simulink model "ZOP_Main"  (R2018b)
settings: Solver=FixedStepDiscrete  StartTime=0.0  StopTime=inf  FixedStep=0.01  RelTol=1e-3
PostLoadFcn:
  | if any(exist('dsrtsu_mdlpostloadfcn', 'file') ~= 0), dsrtsu_mdlpostloadfcn('Execute', bdroot); end
values from neighbouring files (symbols this model uses):
  k_ZOP_ALC_Ramp = 1.0    [ZOP_Func.sldd]
  k_ZOP_LS_ChangingDist = 5.0    [ZOP_Func.sldd]
  k_ZOP_LS_ChangingTime = 0.5    [ZOP_Func.sldd]
  k_ZOP_SpdLmt_Enable = 1.0    [ZOP_Func.sldd]
  k_ZOP_V2X_Enable = 1.0    [ZOP_Func.sldd]
  k_ZOP_VcTJA_Enable = 1.0    [ZOP_Func.sldd]
  k_ZOP_VoiceAct_Enable = 1.0    [ZOP_Func.sldd]
  MODE_ZOP_ACTIVE = 3.0    [ZOP_Func.sldd]
  MODE_ZOP_FINISH = 10.0    [ZOP_Func.sldd]
  MODE_ZOP_LC = 7.0    [ZOP_Func.sldd]
(part 1 of 2)
settings Model: DSRTSU_INTERNAL_RTI_VER=540  DSRTSU_INTERNAL_RTI_TYPE=rti1401  RTICANMMDATA=struct('GeneralSetupData',struct('modelroot','F:\DatabaseZO\08.Code\Model\ZOP_Integration','generalsettings',struct('filesettings',struct('destfolder',struct('Name','RTICANMM_FILES','Check',1),'buildfolder',struct('Name','.','Check',1),'AbsDestfolder',struct('Name','F:\DatabaseZO\08.Code\Model\ZOP_Integration\RTICANMM_FILES'),'AbsBuildfolder',struct('Name','F:\DatabaseZO\08.Code\Model\ZOP_Integration'))),'options',struct('addpaths',1,'rmpaths',1,'addtrcexclusion',logical(1),'cannavigator',struct('checkmonitoring',0),'show_usrtrc',0,'use_usrtrc',0),'advanced',struct('options',ones(1,100)),'MPSetup',{{}},'RTI',struct('Type','RTI1401','Ver','7.12','Date','02-May-2019'),'modelname','ZOP_Main','block','ZOP_Main'))  DSRTSU_INTERNAL_RTIFPGA=130  Creator=zjw  LastModifiedBy=zjw
settings OptimizationCC: BlockReduction=off  ConditionallyExecuteInputs=off  DefaultUnderspecifiedDataType=single  BufferReuse=off  EnhancedBackFolding=on  ExpressionFolding=off  PassReuseOutputArgsThreshold=0  LocalBlockOutputs=off  OptimizeBlockOrder=speed  DifferentSizesBufferReuse=on
settings DebuggingCC: ParameterTunabilityLossMsg=error
settings HardwareCC: ProdBitPerPointer=32  ProdBitPerSizeT=32  ProdBitPerPtrDiffT=32  ProdLargestAtomicInteger=Integer  ProdEndianess=BigEndian  ProdWordSize=32  ProdHWDeviceType=Custom Processor->Custom  TargetIntDivRoundTo=Zero  TargetEndianess=BigEndian  TargetHWDeviceType=Custom Processor->Custom
settings ModelReferenceCC: ModelReferenceNumInstancesAllowed=Single
settings SFSimCC: MATLABDynamicMemAlloc=off
settings RTWCC: SystemTargetFile=rti1401.tlc  MakeCommand=make_rti  TemplateMakefile=rti1401.tmf  Description=dSPACE DS1401 Hardware Platform  GenerateReport=on  LaunchReport=on
settings CodeAppCC: OperatorAnnotations=on
settings STFCustomTargetCC: ParMdlRefBuildCompliant=on  SystemTargetFile=rti1401.tlc
settings GRTTargetCC: TargetLangStandard=C89/C90 (ANSI)  CompOptLevelCompliant=off  ConcurrentExecutionCompliant=off  CombineOutputUpdateFcns=off  MatFileLogging=off  CPPClassGenCompliant=off  UseToolchainInfoCompliant=off

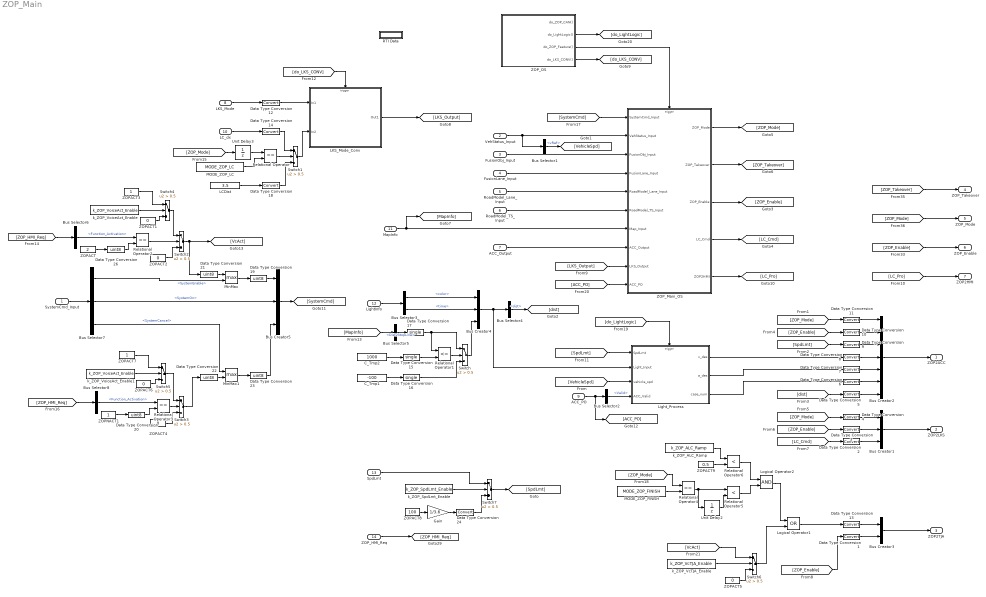
== system ZOP_Main ==
  SystemCmd_Input : Inport  OutDataTypeStr=Bus: SystemCmd_ST  BusOutputAsStruct=on
  VehStatus_Input : Inport  Port=2  OutDataTypeStr=Bus: VSI_VEHSTATE_ST  BusOutputAsStruct=on
  FusionObj_Input : Inport  Port=3  OutDataTypeStr=Bus: FUS_OBJ_OUTPUT_ST  BusOutputAsStruct=on
  FusionLane_Input : Inport  Port=4  OutDataTypeStr=Bus: FUS_LANE_OUTPUT_ST  BusOutputAsStruct=on
  RoadModel_Lane_Input : Inport  Port=5  OutDataTypeStr=Bus: LANEMODEL_OUTPUT_ST  BusOutputAsStruct=on
  RoadModel_TS_Input : Inport  Port=6  OutDataTypeStr=Bus: HWA_TARGETOBJECT_OUTPUT_ST  BusOutputAsStruct=on
  ACC_Output : Inport  Port=7  OutDataTypeStr=Bus: ACC_Status_ST  BusOutputAsStruct=on
  LKS_Mode : Inport  Port=8  BusOutputAsStruct=on
  ACC_PO : Inport  Port=9  OutDataTypeStr=Bus: ATS_PO_ST  BusOutputAsStruct=on
  LC_dx : Inport  Port=10  BusOutputAsStruct=on
  MapInfo : Inport  Port=11  OutDataTypeStr=Bus: MapInfo_ST  BusOutputAsStruct=on
  LightInfo : Inport  Port=12  OutDataTypeStr=Bus: Light_Info_ST  BusOutputAsStruct=on
  SpdLmt : Inport  Port=13  BusOutputAsStruct=on
  ZOP_HMI_Req : Inport  Port=14  OutDataTypeStr=Bus: ZOP_HMI_REQ  BusOutputAsStruct=on
  Bus Creator1 : BusCreator  Inputs=3  OutDataTypeStr=Bus: ZOP2LCK  NonVirtualBus=on
      settings: InheritFromInputs=off
  Bus Creator2 : BusCreator  Inputs=7  OutDataTypeStr=Bus: ZOP2ACC  NonVirtualBus=on
      settings: InheritFromInputs=off
  Bus Creator3 : BusCreator  Inputs=2  OutDataTypeStr=Bus: ZOP2TJA  NonVirtualBus=on
      settings: InheritFromInputs=off
  Bus Creator4 : BusCreator  Inputs=3  OutDataTypeStr=Bus: Light_Info_ST  NonVirtualBus=on
      settings: InheritFromInputs=off
  Bus Creator5 : BusCreator  Inputs=3  OutDataTypeStr=Bus: SystemCmd_ST  NonVirtualBus=on
      settings: InheritFromInputs=off
  Bus Selector1 : BusSelector  OutputSignals=vRef
  Bus Selector2 : BusSelector  OutputSignals=Valid
  Bus Selector3 : BusSelector  OutputSignals=color,time
  Bus Selector4 : BusSelector  OutputSignals=dist
  Bus Selector5 : BusSelector  OutputSignals=Dist2StopLine
  Bus Selector6 : BusSelector  OutputSignals=Function_Activation
  Bus Selector7 : BusSelector  OutputSignals=SystemEnable,SystemOn,SystemCancel
  Bus Selector8 : BusSelector  OutputSignals=Function_Activation
  C_Tmp1 : Constant  Value=-100
  C_Tmp2 : Constant  Value=1000
  Data Type Conversion{1..14,18,24} (16 alike) : DataTypeConversion
  Data Type Conversion15 : DataTypeConversion  OutDataTypeStr=single
  Data Type Conversion16 : DataTypeConversion  OutDataTypeStr=single
  Data Type Conversion17 : DataTypeConversion  OutDataTypeStr=single
  Data Type Conversion{19..23,26} (6 alike) : DataTypeConversion  OutDataTypeStr=uint8
  Gain : Gain  Gain=1/3.6
  LCDist : Constant  Value=3.5
  LKS_Mode_Conv : Subsystem
  Light_Process : Subsystem
  Logical Operator1 : Logic  Operator=OR  AllPortsSameDT=off  OutDataTypeStr=boolean
  Logical Operator2 : Logic  AllPortsSameDT=off  OutDataTypeStr=boolean
  MODE_ZOP_FINISH : Constant  Value=MODE_ZOP_FINISH
  MODE_ZOP_LC : Constant  Value=MODE_ZOP_LC
  MinMax : MinMax  Function=max  Inputs=2
  MinMax1 : MinMax  Function=max  Inputs=2
  RTI Data : Subsystem  Tag=struct('RTIDataServer',struct('RTIDataServerVs','2','RTIModelDescription','struct(''main'',''ZOP_Main'',''sub'','''',''isMp'',0)'))  LoadFcn="if exist('rtidc'), try,  rtidc('DataHostBlockClbLoad', gcbh); catch, disp(['Warning: ''LoadFcn'' for RTI Data block failed: ' lasterr]); end, end,"  mask(RTI_DATA_HOST){}
      mask help:
      | RTI Data Block.
      | This block is used by RTI to store internal model-dependent data.
      | Please keep this block on the root level of the model. Deleting this block will result in data loss.
      |
      | NEVER DELETE OR COPY THIS BLOCK!
      settings: CopyFcn="if exist('rtidc'), try,  rtidc('DataHostBlockClbCopy', gcbh); catch, disp(['Warning: ''CopyFcn'' for RTI Data block failed: ' lasterr]); end, end,"  DeleteFcn="if exist('rtidc'), try,  rtidc('DataHostBlockClbDelete', gcbh); catch, disp(['Warning: ''DeleteFcn'' for RTI Data block failed: ' lasterr]); end, end,"  ModelCloseFcn="if exist('rtidc'), try,  rtidc('DataHostBlockClbModelClose', gcbh); catch, disp(['Warning: ''ModelCloseFcn'' for RTI Data block failed: ' lasterr]); end, end,"  PreSaveFcn="if exist('rtidc'), try,  rtidc('DataHostBlockClbPreSave', gcbh); catch, disp(['Warning: ''PreSaveFcn'' for RTI Data block failed: ' lasterr]); end, end,"  PostSaveFcn="if exist('rtidc'), try,  rtidc('DataHostBlockClbPostSave', gcbh); catch, disp(['Warning: ''PostSaveFcn'' for RTI Data block failed: ' lasterr]); end, end,"  NameChangeFcn="if exist('rtidc'), try,  rtidc('DataHostBlockClbNameChange', gcbh); catch, disp(['Warning: ''NameChangeFcn'' for RTI Data block failed: ' lasterr]); end, end,"
      mask Help:
      | RTI Data Block.
      | This block is used by RTI to store internal model-dependent data.
      | Please keep this block on the root level of the model. Deleting this block will result in data loss.
      | 
      | NEVER DELETE OR COPY THIS BLOCK!
      mask Display:
      | text(0.5, 0.5, 'RTI Data', 'HorizontalAlignment', 'center');
      | plot([1 0]);
  Relational Operator{,2..4} (4 alike) : RelationalOperator  Operator===  OutDataTypeStr=boolean  RndMeth=Simplest
  Relational Operator1 : RelationalOperator  Operator=<=  OutDataTypeStr=boolean  RndMeth=Simplest
  Relational Operator5 : RelationalOperator  Operator=<  OutDataTypeStr=boolean  RndMeth=Simplest
  Relational Operator6 : RelationalOperator  Operator=<  OutDataTypeStr=boolean  RndMeth=Simplest
  Switch{,1..7} (8 alike) : Switch  Criteria=u2 > Threshold  Threshold=0.5
  Unit Delay2 : UnitDelay  SampleTime=-1
  Unit Delay3 : UnitDelay  SampleTime=-1
  ZOPACT : Constant  Value=2
  ZOPACT{1..2,4..6} (5 alike) : Constant  Value=0
  ZOPACT3 : Constant
  ZOPACT7 : Constant
  ZOPACT8 : Constant  Value=100
  ZOPACT9 : Constant  Value=0.5
  ZOPNACT1 : Constant
  ZOP_Main_OS : Subsystem
  ZOP_OS : Stateflow chart  TreatAsAtomicUnit=on
  k_ZOP_ALC_Ramp : Constant  Value=k_ZOP_ALC_Ramp
  k_ZOP_SpdLmt_Enable : Constant  Value=k_ZOP_SpdLmt_Enable
  k_ZOP_VcTJA_Enable : Constant  Value=k_ZOP_VcTJA_Enable
  k_ZOP_VoiceAct_Enable : Constant  Value=k_ZOP_VoiceAct_Enable
  k_ZOP_VoiceAct_Enable1 : Constant  Value=k_ZOP_VoiceAct_Enable
  ZOP2ACC : Outport  OutDataTypeStr=Bus: ZOP2ACC
  ZOP2LKS : Outport  Port=2  OutDataTypeStr=Bus: ZOP2LCK
  ZOP2TJA : Outport  Port=3  OutDataTypeStr=Bus: ZOP2TJA
  ZOP_Takeover : Outport  Port=4
  ZOP_Mode : Outport  Port=5
  ZOP_Enable : Outport  Port=6
  ZOP2HMI : Outport  Port=7  OutDataTypeStr=Bus: ZOP2HMI
  wires:
  ZOP_OS/3(do_ZOP_Feature()) -> ZOP_Main_OS/Trigger
  ZOP_Main_OS/1(ZOP_Mode) -> [ZOP_Mode]
  ZOP_Main_OS/2(ZOP_Takeover) -> [ZOP_Takeover]
  MapInfo/1 -> [MapInfo], ZOP_Main_OS/7(Map_Input)
  ZOP_OS/2(do_LightLogic()) -> [do_LightLogic]
  [do_LightLogic] -> Light_Process/Trigger
  VehStatus_Input/1 -> Bus Selector1/1, ZOP_Main_OS/2(VehStatus_Input)
  FusionObj_Input/1 -> ZOP_Main_OS/3(FusionObj_Input)
  FusionLane_Input/1 -> ZOP_Main_OS/4(FusionLane_Input)
  RoadModel_Lane_Input/1 -> ZOP_Main_OS/5(RoadModel_Lane_Input)
  RoadModel_TS_Input/1 -> ZOP_Main_OS/6(RoadModel_TS_Input)
  Bus Selector1/1 -> [VehicleSpd]  "<vRef>"
  [VehicleSpd] -> Light_Process/3(vehicle_spd)
  ACC_PO/1 -> [ACC_PO], Bus Selector2/1
  Bus Selector2/1 -> Light_Process/4(ACC_Valid)  "<Valid>"
  [ZOP_Mode] -> Data Type Conversion11/1
  [SpdLmt] -> Data Type Conversion9/1
  Bus Selector4/1 -> [dist]  "<dist>"
  Light_Process/1(v_des) -> Data Type Conversion8/1
  ZOP_Main_OS/3(ZOP_Enable) -> [ZOP_Enable]
  [ZOP_Enable] -> Data Type Conversion10/1
  [ZOP_Mode] -> Data Type Conversion4/1
  [ZOP_Enable] -> Data Type Conversion3/1
  ZOP_Main_OS/4(LC_Cmd) -> [LC_Cmd]
  [LC_Cmd] -> Data Type Conversion2/1
  Light_Process/2(a_des) -> Data Type Conversion7/1
  [dist] -> Data Type Conversion5/1
  Light_Process/3(case_num) -> Data Type Conversion6/1
  Data Type Conversion13/1 -> Bus Creator3/1
  [ZOP_Enable] -> Data Type Conversion1/1
  ACC_Output/1 -> ZOP_Main_OS/8(ACC_Output)
  [LKS_Output] -> ZOP_Main_OS/9(LKS_Output)
  Data Type Conversion1/1 -> Bus Creator3/2
  Data Type Conversion2/1 -> Bus Creator1/3
  Data Type Conversion3/1 -> Bus Creator1/2
  Data Type Conversion4/1 -> Bus Creator1/1
  Data Type Conversion5/1 -> Bus Creator2/7
  Data Type Conversion6/1 -> Bus Creator2/6
  Data Type Conversion7/1 -> Bus Creator2/5
  Data Type Conversion8/1 -> Bus Creator2/4
  Data Type Conversion9/1 -> Bus Creator2/3
  Data Type Conversion10/1 -> Bus Creator2/2
  Data Type Conversion11/1 -> Bus Creator2/1
  [SpdLmt] -> Light_Process/1(SpdLmt)
  LKS_Mode/1 -> Data Type Conversion12/1
  LC_dx/1 -> Data Type Conversion14/1
  LKS_Mode_Conv/1(Out1) -> [LKS_Output]
  ZOP_OS/4(do_LKS_CONV()) -> [do_LKS_CONV]
  [do_LKS_CONV] -> LKS_Mode_Conv/Trigger
  [ZOP_Takeover] -> ZOP_Takeover/1
  [ZOP_Mode] -> ZOP_Mode/1
  [ZOP_Enable] -> ZOP_Enable/1
  Data Type Conversion12/1 -> LKS_Mode_Conv/1(In1)
  Bus Creator2/1 -> ZOP2ACC/1
  Bus Creator1/1 -> ZOP2LKS/1
  Bus Creator3/1 -> ZOP2TJA/1
  LightInfo/1 -> Bus Selector3/1
  Bus Selector3/1 -> Bus Creator4/1  "<color>"
  Bus Selector3/2 -> Bus Creator4/2  "<time>"
  Bus Creator4/1 -> Light_Process/2(Light_Input), Bus Selector4/1
  Relational Operator1/1 -> Switch/2
  C_Tmp1/1 -> Data Type Conversion16/1
  Switch/1 -> Bus Creator4/3
  C_Tmp2/1 -> Data Type Conversion15/1
  Data Type Conversion15/1 -> Relational Operator1/2
  Data Type Conversion16/1 -> Switch/3
  ZOP_Main_OS/5(ZOP2HMI) -> [LC_Pro]
  [LC_Pro] -> ZOP2HMI/1
  [MapInfo] -> Bus Selector5/1
  Bus Selector5/1 -> Data Type Conversion17/1  "<Dist2StopLine>"
  Data Type Conversion17/1 -> Relational Operator1/1, Switch/1
  [ZOP_Mode] -> Unit Delay3/1
  MODE_ZOP_LC/1 -> Relational Operator/2
  Relational Operator/1 -> Switch1/2
  Switch1/1 -> LKS_Mode_Conv/2(In2)
  Data Type Conversion14/1 -> Switch1/1
  LCDist/1 -> Data Type Conversion18/1
  Unit Delay3/1 -> Relational Operator/1
  Data Type Conversion18/1 -> Switch1/3
  ZOP_HMI_Req/1 -> [ZOP_HMI_Req]
  [ZOP_HMI_Req] -> Bus Selector6/1
  SystemCmd_Input/1 -> Bus Selector7/1
  Bus Selector6/1 -> Relational Operator2/1  "<Function_Activation>"
  ZOPACT/1 -> Data Type Conversion26/1
  Data Type Conversion26/1 -> Relational Operator2/2
  Bus Selector7/1 -> MinMax/2  "<SystemEnable>"
  Bus Selector7/3 -> MinMax1/1  "<SystemCancel>"
  Data Type Conversion19/1 -> Bus Creator5/1
  MinMax/1 -> Data Type Conversion19/1
  Data Type Conversion20/1 -> Relational Operator3/2
  ZOPNACT1/1 -> Data Type Conversion20/1
  Bus Selector8/1 -> Relational Operator3/1  "<Function_Activation>"
  [ZOP_HMI_Req] -> Bus Selector8/1
  Relational Operator2/1 -> Switch2/2
  ZOPACT2/1 -> Switch2/3
  ZOPACT4/1 -> Switch3/3
  Switch2/1 -> Data Type Conversion21/1, [VcAct]
  Data Type Conversion21/1 -> MinMax/1
  Relational Operator3/1 -> Switch3/2
  Switch3/1 -> Data Type Conversion22/1
  Data Type Conversion22/1 -> MinMax1/2
  MinMax1/1 -> Data Type Conversion23/1
  Bus Creator5/1 -> [SystemCmd]
  [SystemCmd] -> ZOP_Main_OS/1(SystemCmd_Input)
  MODE_ZOP_FINISH/1 -> Relational Operator4/2
  [ZOP_Mode] -> Relational Operator4/1
  Bus Selector7/2 -> Bus Creator5/2  "<SystemOn>"
  Data Type Conversion23/1 -> Bus Creator5/3
  [ACC_PO] -> ZOP_Main_OS/10(ACC_PO)
  k_ZOP_VoiceAct_Enable/1 -> Switch4/2
  ZOPACT3/1 -> Switch4/1
  ZOPACT1/1 -> Switch4/3
  Switch4/1 -> Switch2/1
  ZOPACT6/1 -> Switch5/3
  k_ZOP_VoiceAct_Enable1/1 -> Switch5/2
  ZOPACT7/1 -> Switch5/1
  Switch5/1 -> Switch3/1
  Logical Operator1/1 -> Data Type Conversion13/1
  Switch6/1 -> Logical Operator1/2
  k_ZOP_VcTJA_Enable/1 -> Switch6/2
  ZOPACT5/1 -> Switch6/3
  [VcAct] -> Switch6/1
  SpdLmt/1 -> Switch7/1
  ZOPACT8/1 -> Gain/1
  k_ZOP_SpdLmt_Enable/1 -> Switch7/2
  Switch7/1 -> [SpdLmt]
  Gain/1 -> Data Type Conversion24/1
  Data Type Conversion24/1 -> Switch7/3
  Relational Operator4/1 -> Unit Delay2/1, Relational Operator5/1
  Unit Delay2/1 -> Relational Operator5/2
  Logical Operator2/1 -> Logical Operator1/1
  Relational Operator5/1 -> Logical Operator2/2
  Relational Operator6/1 -> Logical Operator2/1
  k_ZOP_ALC_Ramp/1 -> Relational Operator6/1
  ZOPACT9/1 -> Relational Operator6/2

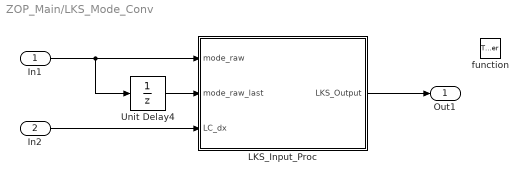
== system ZOP_Main/LKS_Mode_Conv ==
  In1 : Inport
  In2 : Inport  Port=2
  function : TriggerPort  TriggerType=function-call  VariantControl=Variant
  LKS_Input_Proc : MATLAB Function  TreatAsAtomicUnit=on
  Unit Delay4 : UnitDelay  SampleTime=-1
  Out1 : Outport
  wires:
  In1/1 -> LKS_Input_Proc/1(mode_raw), Unit Delay4/1
  Unit Delay4/1 -> LKS_Input_Proc/2(mode_raw_last)
  In2/1 -> LKS_Input_Proc/3(LC_dx)
  LKS_Input_Proc/1(LKS_Output) -> Out1/1

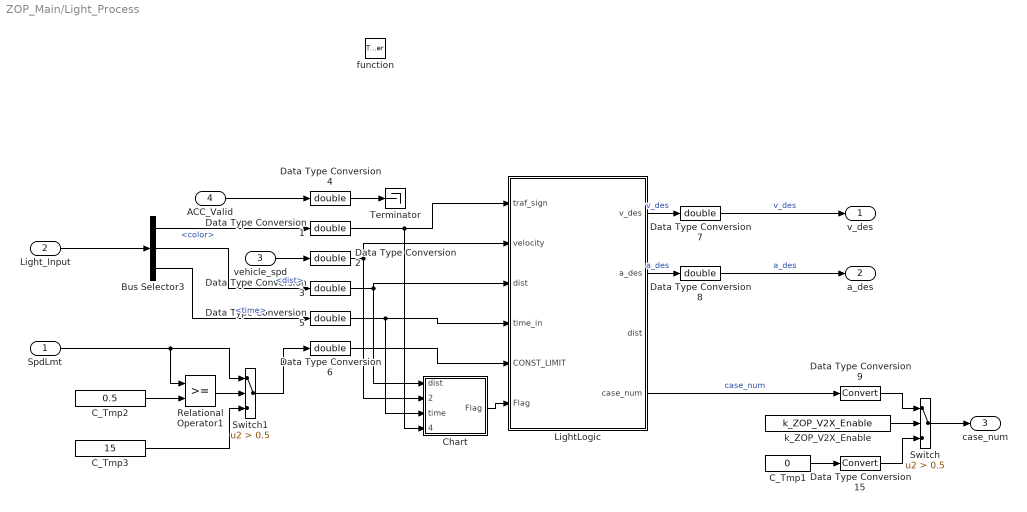
== system ZOP_Main/Light_Process ==
  SpdLmt : Inport  BusOutputAsStruct=on
  Light_Input : Inport  Port=2  OutDataTypeStr=Bus: Light_Info_ST  BusOutputAsStruct=on
  vehicle_spd : Inport  Port=3  BusOutputAsStruct=on
  ACC_Valid : Inport  Port=4  BusOutputAsStruct=on
  function : TriggerPort  TriggerType=function-call  VariantControl=Variant
  Bus Selector3 : BusSelector  OutputSignals=color,dist,time
  C_Tmp1 : Constant  Value=0
  C_Tmp2 : Constant  Value=0.5
  C_Tmp3 : Constant  Value=15
  Chart : Stateflow chart  TreatAsAtomicUnit=on
  Data Type Conversion{1..8} (8 alike) : DataTypeConversion  OutDataTypeStr=double
  Data Type Conversion15 : DataTypeConversion
  Data Type Conversion9 : DataTypeConversion
  LightLogic : MATLAB Function  TreatAsAtomicUnit=on
  Relational Operator1 : RelationalOperator  OutDataTypeStr=boolean  RndMeth=Simplest
  Switch : Switch  Criteria=u2 > Threshold  Threshold=0.5
  Switch1 : Switch  Criteria=u2 > Threshold  Threshold=0.5
  Terminator : Terminator
  k_ZOP_V2X_Enable : Constant  Value=k_ZOP_V2X_Enable
  v_des : Outport
  a_des : Outport  Port=2
  case_num : Outport  Port=3
  wires:
  Relational Operator1/1 -> Switch1/2
  C_Tmp2/1 -> Relational Operator1/2
  C_Tmp3/1 -> Switch1/3
  SpdLmt/1 -> Relational Operator1/1, Switch1/1
  LightLogic/2(a_des) -> Data Type Conversion8/1  "a_des"
  Bus Selector3/2 -> Data Type Conversion3/1  "<dist>"
  Data Type Conversion9/1 -> Switch/1
  Data Type Conversion3/1 -> Chart/1(dist), LightLogic/3("dist ")
  Switch/1 -> case_num/1
  Data Type Conversion1/1 -> Chart/4(traf_sign), LightLogic/1(traf_sign)
  Switch1/1 -> Data Type Conversion6/1
  LightLogic/4(case_num) -> Data Type Conversion9/1  "case_num"
  Data Type Conversion6/1 -> LightLogic/5(CONST_LIMIT)
  Data Type Conversion2/1 -> Chart/2(velocity), LightLogic/2(velocity)
  Bus Selector3/1 -> Data Type Conversion1/1  "<color>"
  Data Type Conversion8/1 -> a_des/1  "a_des"
  Chart/1(Flag) -> LightLogic/6(Flag)
  Bus Selector3/3 -> Data Type Conversion5/1  "<time>"
  ACC_Valid/1 -> Data Type Conversion4/1
  k_ZOP_V2X_Enable/1 -> Switch/2
  Data Type Conversion5/1 -> Chart/3(time), LightLogic/4(time_in)
  Data Type Conversion7/1 -> v_des/1  "v_des"
  C_Tmp1/1 -> Data Type Conversion15/1
  LightLogic/1(v_des) -> Data Type Conversion7/1  "v_des"
  vehicle_spd/1 -> Data Type Conversion2/1
  Data Type Conversion15/1 -> Switch/3
  Data Type Conversion4/1 -> Terminator/1
  Light_Input/1 -> Bus Selector3/1

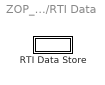
== system ZOP_Main/RTI Data ==
  RTI Data Store : Subsystem  Tag="struct('private',struct('version',struct('dsVer',uint32(2),'dsVerCreation',uint32(2),'RTI',struct('ver','7.12','type','RTI1401')),'access',struct('type','Model','isPerm',1,'created',['30-Dec-2020 11:01:12'],'modified',['10-Mar-2021 09:22:38'],'location','')),'public',struct('main',struct('data',[]),'sub',struct('name',{{'ZOP_Main'}},'data',{{struct('TH',struct('thTaskInfo',struct('taskType',{'TIMER','HWINT','TMRINT','SWINT','GLINT'},'tasksNumOf',{1,0,0,0,0},'srcIds',{{'TIMERA'},{},{},{},{}},'taskNames',{{['Timer Task 1']},{},{},{},{}})),'th_tc',struct('dataType','TASK','taskGroupId','','taskGroupList',{{}},'taskSchedulingPolicy','FCFS','taskType','TIMER','blkh',-1,'srcId','TIMERA','srcSgnName',['Timer A interrupt'],'srcCpuName','','taskName',['Timer Task 1  [0.01] s'],'taskNameDisplayExt','','smplTime',0.01,'smplTimeOffs',0,'hasFixedPriority',0,'priority',1,'hasFixedOvc',0,'ovcType',3,'ovcMax',1),'tc_th',struct('dataType','TASK','taskGroupId','','taskGroupList',{{}},'taskSchedulingPolicy','FCFS','taskType','TIMER','blkh',-1,'srcId','TIMERA','srcSgnName',['Timer A interrupt'],'srcCpuName','','taskName',['Timer Task 1  [0.01] s'],'taskNameDisplayExt','','smplTime',0.01,'smplTimeOffs',0,'hasFixedPriority',0,'priority',1,'hasFixedOvc',0,'ovcType',3,'ovcMax',1))}})))"  mask(RTI_DATA_STORE){}
      mask help:
      | RTI Data Store Block. This block is used by RTI to store internal model dependent data. Deleting this block will result in data loss.
      |
      | NEVER DELETE, COPY, OR MODIFY THIS BLOCK!
      mask Help:
      | RTI Data Store Block. This block is used by RTI to store internal model dependent data. Deleting this block will result in data loss.
      | 
      | NEVER DELETE, COPY, OR MODIFY THIS BLOCK!
      mask Display: text(0.5, 0.5, ' ', 'HorizontalAlignment', 'center');

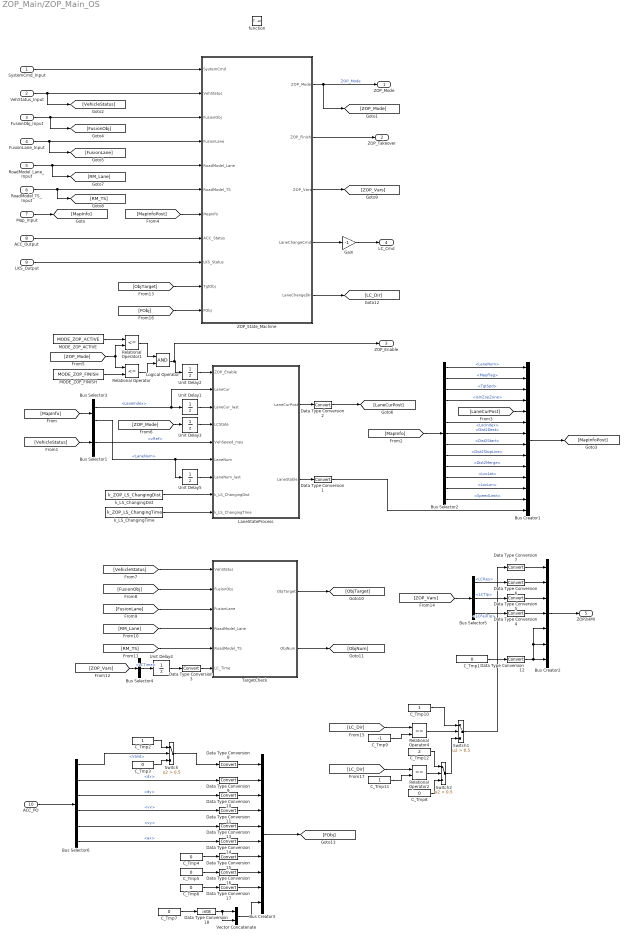
== system ZOP_Main/ZOP_Main_OS ==
  SystemCmd_Input : Inport  OutDataTypeStr=Bus: SystemCmd_ST  BusOutputAsStruct=on
  VehStatus_Input : Inport  Port=2  OutDataTypeStr=Bus: VSI_VEHSTATE_ST  BusOutputAsStruct=on
  FusionObj_Input : Inport  Port=3  OutDataTypeStr=Bus: FUS_OBJ_OUTPUT_ST  BusOutputAsStruct=on
  FusionLane_Input : Inport  Port=4  OutDataTypeStr=Bus: FUS_LANE_OUTPUT_ST  BusOutputAsStruct=on
  RoadModel_Lane_Input : Inport  Port=5  OutDataTypeStr=Bus: LANEMODEL_OUTPUT_ST  BusOutputAsStruct=on
  RoadModel_TS_Input : Inport  Port=6  OutDataTypeStr=Bus: HWA_TARGETOBJECT_OUTPUT_ST  BusOutputAsStruct=on
  Map_Input : Inport  Port=7  OutDataTypeStr=Bus: MapInfo_ST  BusOutputAsStruct=on
  ACC_Output : Inport  Port=8  OutDataTypeStr=Bus: ACC_Status_ST  BusOutputAsStruct=on
  LKS_Output : Inport  Port=9  OutDataTypeStr=Bus: LKS_Status_ST  BusOutputAsStruct=on
  ACC_PO : Inport  Port=10  OutDataTypeStr=Bus: ATS_PO_ST  BusOutputAsStruct=on
  function : TriggerPort  TriggerType=function-call  VariantControl=Variant
  Bus Creator1 : BusCreator  Inputs=14  OutDataTypeStr=Bus: MapInfo_ST_Post  NonVirtualBus=on
      settings: InheritFromInputs=off
  Bus Creator2 : BusCreator  Inputs=7  OutDataTypeStr=Bus: ZOP2HMI  NonVirtualBus=on
      settings: InheritFromInputs=off
  Bus Creator3 : BusCreator  Inputs=10  OutDataTypeStr=Bus: ZOP_Object_ST  NonVirtualBus=on
      settings: InheritFromInputs=off
  Bus Selector1 : BusSelector  OutputSignals=vRef
  Bus Selector2 : BusSelector  OutputSignals=LaneNum,MapFlag,TgtSpd,isInZopZone,LaneIndex,LocIndex,Dist2Dest,Dist2Start,Dist2StopLine,Dist2Merge,LocLat,LocLon,SpeedLimit
  Bus Selector3 : BusSelector  OutputSignals=LaneIndex,LaneNum
  Bus Selector4 : BusSelector  OutputSignals=LCTime
  Bus Selector5 : BusSelector  OutputSignals=LCRes,LCTip,LCFailTip
  Bus Selector6 : BusSelector  OutputSignals=Valid,dx,dy,vx,vy,ax
  C_Tmp{1,3..8} (7 alike) : Constant  Value=0
  C_Tmp10 : Constant
  C_Tmp11 : Constant
  C_Tmp12 : Constant  Value=2
  C_Tmp2 : Constant
  C_Tmp9 : Constant  Value=-1
  Data Type Conversion{1..17} (17 alike) : DataTypeConversion
  Data Type Conversion18 : DataTypeConversion  OutDataTypeStr=int8
  Gain : Gain  Gain=-1
  LaneStateProcess : Stateflow chart  TreatAsAtomicUnit=on
  Logical Operator : Logic  AllPortsSameDT=off  OutDataTypeStr=boolean
  MODE_ZOP_ACTIVE : Constant  Value=MODE_ZOP_ACTIVE
  MODE_ZOP_FINISH : Constant  Value=MODE_ZOP_FINISH
  Relational Operator : RelationalOperator  Operator=<=  OutDataTypeStr=boolean  RndMeth=Simplest
  Relational Operator1 : RelationalOperator  Operator=<=  OutDataTypeStr=boolean  RndMeth=Simplest
  Relational Operator2 : RelationalOperator  Operator===  OutDataTypeStr=boolean  RndMeth=Simplest
  Relational Operator4 : RelationalOperator  Operator===  OutDataTypeStr=boolean  RndMeth=Simplest
  Switch : Switch  Criteria=u2 > Threshold  Threshold=0.5
  Switch1 : Switch  Criteria=u2 > Threshold  Threshold=0.5
  Switch2 : Switch  Criteria=u2 > Threshold  Threshold=0.5
  TargetCheck : Stateflow chart  TreatAsAtomicUnit=on
  Unit Delay{1..5} (5 alike) : UnitDelay  SampleTime=-1
  Vector Concatenate : Concatenate
  ZOP_State_Machine : Stateflow chart  TreatAsAtomicUnit=on
  k_LS_ChangingDist : Constant  Value=k_ZOP_LS_ChangingDist
  k_LS_ChangingTime : Constant  Value=k_ZOP_LS_ChangingTime
  ZOP_Mode : Outport
  ZOP_Takeover : Outport  Port=2
  ZOP_Enable : Outport  Port=3
  LC_Cmd : Outport  Port=4
  ZOP2HMI : Outport  Port=5  OutDataTypeStr=Bus: ZOP2HMI
  wires:
  SystemCmd_Input/1 -> ZOP_State_Machine/1(SystemCmd)
  VehStatus_Input/1 -> [VehicleStatus], ZOP_State_Machine/2(VehStatus)
  FusionObj_Input/1 -> [FusionObj], ZOP_State_Machine/3(FusionObj)
  FusionLane_Input/1 -> [FusionLane], ZOP_State_Machine/4(FusionLane)
  RoadModel_Lane_Input/1 -> [RM_Lane], ZOP_State_Machine/5(RoadModel_Lane)
  RoadModel_TS_Input/1 -> [RM_TS], ZOP_State_Machine/6(RoadModel_TS)
  Map_Input/1 -> [MapInfo]
  ACC_Output/1 -> ZOP_State_Machine/8(ACC_Status)
  LKS_Output/1 -> ZOP_State_Machine/9(LKS_Status)
  ZOP_State_Machine/3(ZOP_Vars) -> [ZOP_Vars]
  ZOP_State_Machine/1(ZOP_Mode) -> ZOP_Mode/1, [ZOP_Mode]  "ZOP_Mode"
  ZOP_State_Machine/2(ZOP_Finish) -> ZOP_Takeover/1
  Bus Selector3/1 -> LaneStateProcess/2(LaneCur), Unit Delay1/1  "<LaneIndex>"
  Unit Delay1/1 -> LaneStateProcess/3(LaneCur_last)
  Unit Delay2/1 -> LaneStateProcess/1(ZOP_Enable)
  Unit Delay5/1 -> LaneStateProcess/7(LaneNum_last)
  Data Type Conversion2/1 -> [LaneCurPost]
  Bus Selector3/2 -> Unit Delay5/1, LaneStateProcess/6(LaneNum)  "<LaneNum>"
  Bus Selector1/1 -> LaneStateProcess/5(VehSpeed_mps)  "<vRef>"
  LaneStateProcess/1(LaneCurPost) -> Data Type Conversion2/1
  LaneStateProcess/2(LaneStable) -> Data Type Conversion1/1
  k_LS_ChangingDist/1 -> LaneStateProcess/8(k_LS_ChangingDist)
  [MapInfo] -> Bus Selector3/1
  [VehicleStatus] -> Bus Selector1/1
  k_LS_ChangingTime/1 -> LaneStateProcess/9(k_LS_ChangingTime)
  Bus Creator1/1 -> [MapInfoPost]
  [MapInfo] -> Bus Selector2/1
  [MapInfoPost] -> ZOP_State_Machine/7(MapInfo)
  [ZOP_Mode] -> Relational Operator1/2, Relational Operator/1
  MODE_ZOP_FINISH/1 -> Relational Operator/2
  MODE_ZOP_ACTIVE/1 -> Relational Operator1/1
  Relational Operator1/1 -> Logical Operator/1
  Relational Operator/1 -> Logical Operator/2
  Logical Operator/1 -> ZOP_Enable/1, Unit Delay2/1
  [ZOP_Mode] -> Unit Delay3/1
  Unit Delay3/1 -> LaneStateProcess/4(LCState)
  [VehicleStatus] -> TargetCheck/1(VehStatus)
  [FusionObj] -> TargetCheck/2(FusionObj)
  [FusionLane] -> TargetCheck/3(FusionLane)
  [RM_Lane] -> TargetCheck/4(RoadModel_Lane)
  [RM_TS] -> TargetCheck/5(RoadModel_TS)
  [ZOP_Vars] -> Bus Selector4/1
  Bus Selector4/1 -> Unit Delay4/1  "<LCTime>"
  TargetCheck/1(ObjTarget) -> [ObjTarget]
  [ObjTarget] -> ZOP_State_Machine/10(TgtObj)
  TargetCheck/2(ObjNum) -> [ObjNum]
  Unit Delay4/1 -> Data Type Conversion3/1
  ZOP_State_Machine/4(LaneChangeCmd) -> Gain/1
  Gain/1 -> LC_Cmd/1
  Data Type Conversion3/1 -> TargetCheck/6(LC_Time)
  ZOP_State_Machine/5(LaneChangeDir) -> [LC_Dir]
  Bus Selector2/1 -> Bus Creator1/1  "<LaneNum>"
  Bus Selector2/2 -> Bus Creator1/2  "<MapFlag>"
  Bus Selector2/3 -> Bus Creator1/3  "<TgtSpd>"
  Bus Selector2/4 -> Bus Creator1/4  "<isInZopZone>"
  Bus Selector2/6 -> Bus Creator1/6  "<LocIndex>"
  Bus Selector2/7 -> Bus Creator1/7  "<Dist2Dest>"
  Bus Selector2/8 -> Bus Creator1/8  "<Dist2Start>"
  Bus Selector2/9 -> Bus Creator1/9  "<Dist2StopLine>"
  Bus Selector2/10 -> Bus Creator1/10  "<Dist2Merge>"
  Bus Selector2/11 -> Bus Creator1/11  "<LocLat>"
  Bus Selector2/12 -> Bus Creator1/12  "<LocLon>"
  Bus Selector2/13 -> Bus Creator1/13  "<SpeedLimit>"
  [LaneCurPost] -> Bus Creator1/5
  Data Type Conversion1/1 -> Bus Creator1/14
  [ZOP_Vars] -> Bus Selector5/1
  Switch1/1 -> Data Type Conversion7/1
  Bus Selector5/1 -> Data Type Conversion6/1  "<LCRes>"
  Bus Selector5/3 -> Data Type Conversion4/1  "<LCFailTip>"
  Bus Creator2/1 -> ZOP2HMI/1
  C_Tmp1/1 -> Data Type Conversion12/1
  Data Type Conversion12/1 -> Bus Creator2/6, Bus Creator2/5, Bus Creator2/7
  Bus Selector5/2 -> Data Type Conversion5/1  "<LCTip>"
  Data Type Conversion4/1 -> Bus Creator2/4
  Data Type Conversion5/1 -> Bus Creator2/3
  Data Type Conversion6/1 -> Bus Creator2/2
  Data Type Conversion7/1 -> Bus Creator2/1
  ACC_PO/1 -> Bus Selector6/1
  Bus Selector6/2 -> Data Type Conversion9/1  "<dx>"
  Bus Selector6/3 -> Data Type Conversion10/1  "<dy>"
  Bus Selector6/4 -> Data Type Conversion11/1  "<vx>"
  Bus Selector6/5 -> Data Type Conversion13/1  "<vy>"
  Bus Selector6/6 -> Data Type Conversion14/1  "<ax>"
  Data Type Conversion8/1 -> Bus Creator3/1
  Data Type Conversion9/1 -> Bus Creator3/2
  Data Type Conversion10/1 -> Bus Creator3/3
  Data Type Conversion11/1 -> Bus Creator3/4
  Data Type Conversion13/1 -> Bus Creator3/5
  Data Type Conversion14/1 -> Bus Creator3/6
  Bus Selector6/1 -> Switch/2  "<Valid>"
  C_Tmp3/1 -> Switch/3
  C_Tmp2/1 -> Switch/1
  Switch/1 -> Data Type Conversion8/1
  [FObj] -> ZOP_State_Machine/11(FObj)
  Bus Creator3/1 -> [FObj]
  Data Type Conversion15/1 -> Bus Creator3/7
  C_Tmp4/1 -> Data Type Conversion15/1
  C_Tmp5/1 -> Data Type Conversion16/1
  Data Type Conversion16/1 -> Bus Creator3/8
  C_Tmp6/1 -> Data Type Conversion17/1
  Data Type Conversion17/1 -> Bus Creator3/9
  C_Tmp7/1 -> Data Type Conversion18/1
  Data Type Conversion18/1 -> Vector Concatenate/2, Vector Concatenate/1
  Vector Concatenate/1 -> Bus Creator3/10
  [LC_Dir] -> Relational Operator4/1
  C_Tmp9/1 -> Relational Operator4/2
  Relational Operator4/1 -> Switch1/2
  C_Tmp10/1 -> Switch1/1
  C_Tmp11/1 -> Relational Operator2/2
  [LC_Dir] -> Relational Operator2/1
  Relational Operator2/1 -> Switch2/2
  C_Tmp8/1 -> Switch2/3
  C_Tmp12/1 -> Switch2/1
  Switch2/1 -> Switch1/3

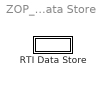
== system ZOP_Main/RTI Data/RTI Data Store ==
  RTI Data Store : Subsystem  mask(RTI_DATA_STORE){}
      mask help:
      | RTI Data Store Block. This block is used by RTI to store internal model dependent data. Deleting this block will result in data loss.
      |
      | NEVER DELETE, COPY, OR MODIFY THIS BLOCK!
      mask Help:
      | RTI Data Store Block. This block is used by RTI to store internal model dependent data. Deleting this block will result in data loss.
      | 
      | NEVER DELETE, COPY, OR MODIFY THIS BLOCK!
      mask Display: text(0.5, 0.5, ' ', 'HorizontalAlignment', 'center');

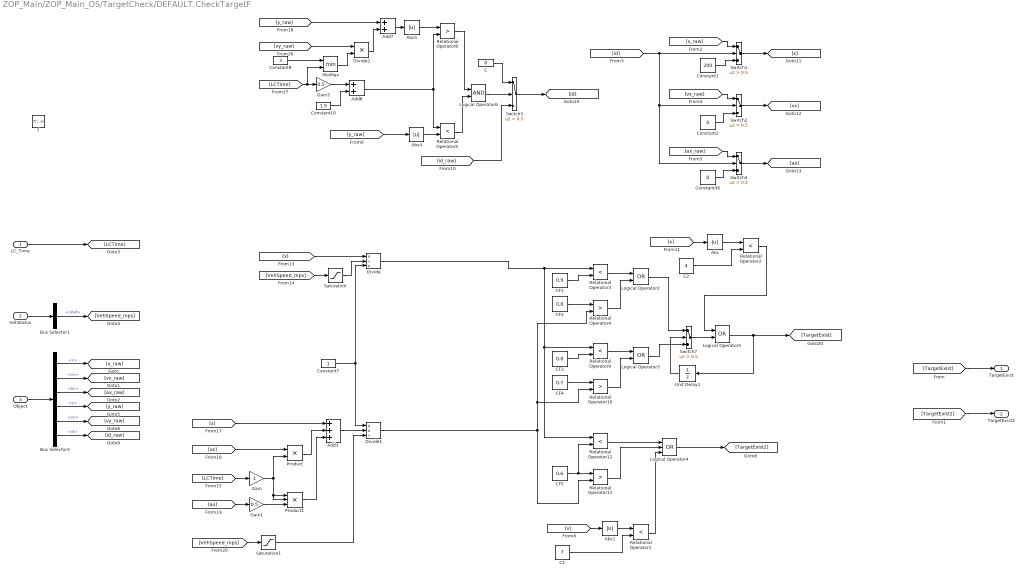
== system ZOP_Main/ZOP_Main_OS/TargetCheck/DEFAULT.CheckTargetF ==
  LC_Time : Inport  OutDataTypeStr=double
  VehStatus : Inport  Port=2  OutDataTypeStr=Bus: VSI_VEHSTATE_ST
  Object : Inport  Port=3  OutDataTypeStr=Bus: ZOP_Object_ST
  f : TriggerPort  TriggerType=function-call  VariantControl=(inherit)
      settings: CopyFcn=Stateflow.SLINSF.SimulinkMan.removeBlockPreDeleteFcn  PreDeleteFcn=Stateflow.SLINSF.SimulinkMan.unsafePredeleteFcn
  Abs{,1,4..5} (4 alike) : Abs
  Add3 : Sum  Inputs=+++
  Add6 : Sum
  Add7 : Sum
  Bus Selector1 : BusSelector  OutputSignals=vRef
  Bus Selector3 : BusSelector  OutputSignals=x,vx,ax,y,vy,id
  C : Constant  Value=0
  C1 : Constant  Value=7
  C2 : Constant  Value=4
  CF1 : Constant  Value=0.9
  CF2 : Constant  Value=0.8
  CF3 : Constant  Value=0.8
  CF4 : Constant  Value=0.7
  CF5 : Constant  Value=0.6
  Constant1 : Constant  Value=200
  Constant10 : Constant  Value=1.5
  Constant2 : Constant  Value=0
  Constant36 : Constant  Value=0
  Constant7 : Constant
  Constant9 : Constant  Value=3
  Divide : Product  Inputs=*/*
  Divide1 : Product  Inputs=**/
  Divide2 : Product  Inputs=**
  Gain : Gain
  Gain1 : Gain  Gain=0.5
  Gain3 : Gain  Gain=0.5
  Logical Operator2 : Logic  Operator=OR  AllPortsSameDT=off  OutDataTypeStr=boolean
  Logical Operator3 : Logic  Operator=OR  AllPortsSameDT=off  OutDataTypeStr=boolean
  Logical Operator4 : Logic  Operator=OR  Inputs=3  AllPortsSameDT=off  OutDataTypeStr=boolean
  Logical Operator5 : Logic  Operator=OR  AllPortsSameDT=off  OutDataTypeStr=boolean
  Logical Operator6 : Logic  AllPortsSameDT=off  OutDataTypeStr=boolean
  MinMax : MinMax  Inputs=2
  Product : Product
  Product1 : Product  Inputs=3
  Relational Operator{1..3,5,9,12} (6 alike) : RelationalOperator  Operator=<  RndMeth=Nearest
  Relational Operator{4,8,10..11} (4 alike) : RelationalOperator  Operator=>  RndMeth=Nearest
  Saturation : Saturate  UpperLimit=100  LowerLimit=0.1
  Saturation1 : Saturate  UpperLimit=100  LowerLimit=0.1
  Switch{1..4,7} (5 alike) : Switch  Criteria=u2 > Threshold  Threshold=0.5
  Unit Delay1 : UnitDelay  SampleTime=-1
  TargetExist : Outport
  TargetExist2 : Outport  Port=2
  wires:
  Abs1/1 -> Relational Operator1/1
  C1/1 -> Relational Operator1/2
  CF1/1 -> Relational Operator3/2
  Relational Operator1/1 -> Logical Operator4/3
  Relational Operator2/1 -> Logical Operator5/1
  [vx] -> Product/1
  [x] -> Abs/1
  [x] -> Abs1/1
  Switch7/1 -> Logical Operator5/2
  [ax] -> Gain1/1
  Logical Operator3/1 -> Switch7/3
  Logical Operator2/1 -> Switch7/1
  Relational Operator11/1 -> Logical Operator4/2
  Relational Operator10/1 -> Logical Operator3/2
  Gain1/1 -> Product1/3
  Divide1/1 -> Relational Operator11/2, Relational Operator4/2, Relational Operator10/2
  Relational Operator9/1 -> Logical Operator3/1
  Logical Operator4/1 -> [TargetExist2]
  Product1/1 -> Add3/3
  Add3/1 -> Divide1/2
  CF5/1 -> Relational Operator11/1, Relational Operator12/2
  Relational Operator3/1 -> Logical Operator2/1
  CF4/1 -> Relational Operator10/1
  [LCTime] -> Gain/1
  Unit Delay1/1 -> Switch7/2
  [x] -> Divide/1
  Constant7/1 -> Divide/3, Divide1/1
  C2/1 -> Relational Operator2/2
  Logical Operator5/1 -> [TargetExist], Unit Delay1/1
  [x] -> Add3/1
  [VehSpeed_mps] -> Saturation1/1
  Product/1 -> Add3/2
  Abs/1 -> Relational Operator2/1
  CF3/1 -> Relational Operator9/2
  CF2/1 -> Relational Operator4/1
  Relational Operator4/1 -> Logical Operator2/2
  Divide/1 -> Relational Operator12/1, Relational Operator9/1, Relational Operator3/1
  Gain/1 -> Product1/2, Product1/1, Product/2
  Saturation1/1 -> Divide1/3
  Relational Operator12/1 -> Logical Operator4/1
  Saturation/1 -> Divide/2
  [VehSpeed_mps] -> Saturation/1
  [TargetExist] -> TargetExist/1
  [TargetExist2] -> TargetExist2/1
  Object/1 -> Bus Selector3/1
  Bus Selector3/1 -> [x_raw]  "<x>"
  Bus Selector3/2 -> [vx_raw]  "<vx>"
  Bus Selector3/3 -> [ax_raw]  "<ax>"
  LC_Time/1 -> [LCTime]
  VehStatus/1 -> Bus Selector1/1
  Bus Selector1/1 -> [VehSpeed_mps]  "<vRef>"
  [id_raw] -> Switch3/3
  Relational Operator5/1 -> Logical Operator6/2
  [y_raw] -> Add7/1
  [LCTime] -> MinMax/2, Gain3/1
  Gain3/1 -> Add6/1
  [y_raw] -> Abs4/1
  Abs4/1 -> Relational Operator5/2
  Relational Operator8/1 -> Logical Operator6/1
  Constant9/1 -> MinMax/1
  MinMax/1 -> Divide2/2
  Divide2/1 -> Add7/2
  Abs5/1 -> Relational Operator8/1
  [vy_raw] -> Divide2/1
  Add6/1 -> Relational Operator5/1, Relational Operator8/2
  Constant10/1 -> Add6/2
  Switch3/1 -> [id]
  Add7/1 -> Abs5/1
  C/1 -> Switch3/1
  [x_raw] -> Switch1/1
  [id] -> Switch2/2, Switch4/2, Switch1/2
  [vx_raw] -> Switch2/1
  [ax_raw] -> Switch4/1
  Constant2/1 -> Switch2/3
  Constant36/1 -> Switch4/3
  Constant1/1 -> Switch1/3
  Bus Selector3/4 -> [y_raw]  "<y>"
  Bus Selector3/5 -> [vy_raw]  "<vy>"
  Logical Operator6/1 -> Switch3/2
  Bus Selector3/6 -> [id_raw]  "<id>"
  Switch1/1 -> [x]
  Switch2/1 -> [vx]
  Switch4/1 -> [ax]

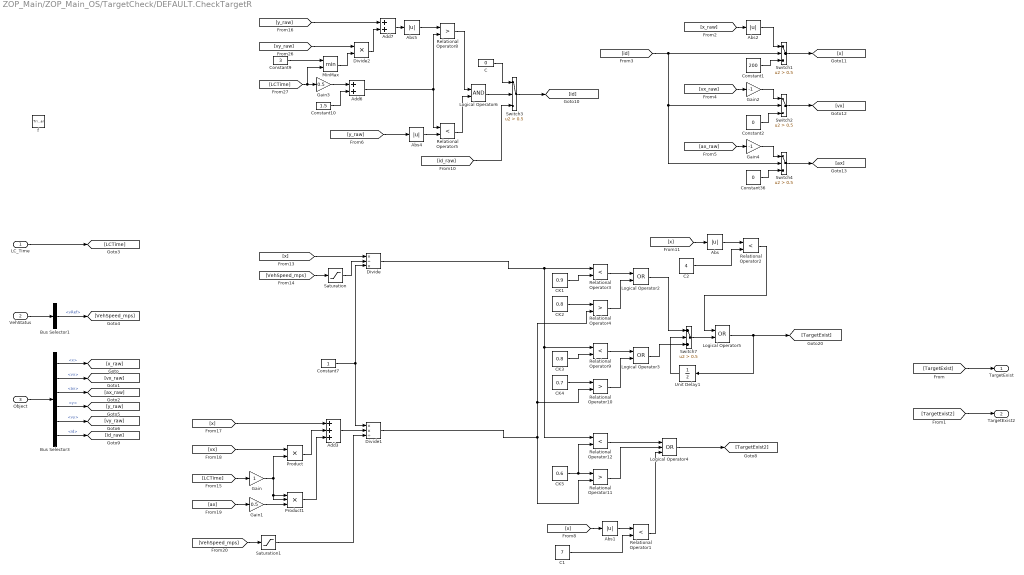
== system ZOP_Main/ZOP_Main_OS/TargetCheck/DEFAULT.CheckTargetR ==
  LC_Time : Inport  OutDataTypeStr=double
  VehStatus : Inport  Port=2  OutDataTypeStr=Bus: VSI_VEHSTATE_ST
  Object : Inport  Port=3  OutDataTypeStr=Bus: ZOP_Object_ST
  f : TriggerPort  TriggerType=function-call  VariantControl=(inherit)
      settings: CopyFcn=Stateflow.SLINSF.SimulinkMan.removeBlockPreDeleteFcn  PreDeleteFcn=Stateflow.SLINSF.SimulinkMan.unsafePredeleteFcn
  Abs{,1..2,4..5} (5 alike) : Abs
  Add3 : Sum  Inputs=+++
  Add6 : Sum
  Add7 : Sum
  Bus Selector1 : BusSelector  OutputSignals=vRef
  Bus Selector3 : BusSelector  OutputSignals=x,vx,ax,y,vy,id
  C : Constant  Value=0
  C1 : Constant  Value=7
  C2 : Constant  Value=4
  CK1 : Constant  Value=0.9
  CK2 : Constant  Value=0.8
  CK3 : Constant  Value=0.8
  CK4 : Constant  Value=0.7
  CK5 : Constant  Value=0.6
  Constant1 : Constant  Value=200
  Constant10 : Constant  Value=1.5
  Constant2 : Constant  Value=0
  Constant36 : Constant  Value=0
  Constant7 : Constant
  Constant9 : Constant  Value=3
  Divide : Product  Inputs=*/*
  Divide1 : Product  Inputs=**/
  Divide2 : Product  Inputs=**
  Gain : Gain
  Gain1 : Gain  Gain=0.5
  Gain2 : Gain  Gain=-1
  Gain3 : Gain  Gain=0.5
  Gain4 : Gain  Gain=-1
  Logical Operator2 : Logic  Operator=OR  AllPortsSameDT=off  OutDataTypeStr=boolean
  Logical Operator3 : Logic  Operator=OR  AllPortsSameDT=off  OutDataTypeStr=boolean
  Logical Operator4 : Logic  Operator=OR  Inputs=3  AllPortsSameDT=off  OutDataTypeStr=boolean
  Logical Operator5 : Logic  Operator=OR  AllPortsSameDT=off  OutDataTypeStr=boolean
  Logical Operator6 : Logic  AllPortsSameDT=off  OutDataTypeStr=boolean
  MinMax : MinMax  Inputs=2
  Product : Product
  Product1 : Product  Inputs=3
  Relational Operator{1..3,5,9,12} (6 alike) : RelationalOperator  Operator=<  RndMeth=Nearest
  Relational Operator{4,8,10..11} (4 alike) : RelationalOperator  Operator=>  RndMeth=Nearest
  Saturation : Saturate  UpperLimit=100  LowerLimit=0.1
  Saturation1 : Saturate  UpperLimit=100  LowerLimit=0.1
  Switch{1..4,7} (5 alike) : Switch  Criteria=u2 > Threshold  Threshold=0.5
  Unit Delay1 : UnitDelay  SampleTime=-1
  TargetExist : Outport
  TargetExist2 : Outport  Port=2
  wires:
  Abs1/1 -> Relational Operator1/1
  C1/1 -> Relational Operator1/2
  CK1/1 -> Relational Operator3/2
  Relational Operator1/1 -> Logical Operator4/3
  Relational Operator2/1 -> Logical Operator5/1
  [vx] -> Product/1
  [x] -> Abs/1
  [x] -> Abs1/1
  Switch7/1 -> Logical Operator5/2
  [ax] -> Gain1/1
  Logical Operator3/1 -> Switch7/3
  Logical Operator2/1 -> Switch7/1
  Relational Operator11/1 -> Logical Operator4/2
  Relational Operator10/1 -> Logical Operator3/2
  Gain1/1 -> Product1/3
  Divide1/1 -> Relational Operator11/2, Relational Operator4/2, Relational Operator10/2
  Relational Operator9/1 -> Logical Operator3/1
  Logical Operator4/1 -> [TargetExist2]
  Product1/1 -> Add3/3
  Add3/1 -> Divide1/2
  CK5/1 -> Relational Operator11/1, Relational Operator12/2
  Relational Operator3/1 -> Logical Operator2/1
  CK4/1 -> Relational Operator10/1
  [LCTime] -> Gain/1
  Unit Delay1/1 -> Switch7/2
  [x] -> Divide/1
  Constant7/1 -> Divide/3, Divide1/1
  C2/1 -> Relational Operator2/2
  Logical Operator5/1 -> [TargetExist], Unit Delay1/1
  [x] -> Add3/1
  [VehSpeed_mps] -> Saturation1/1
  Product/1 -> Add3/2
  Abs/1 -> Relational Operator2/1
  CK3/1 -> Relational Operator9/2
  CK2/1 -> Relational Operator4/1
  Relational Operator4/1 -> Logical Operator2/2
  Divide/1 -> Relational Operator12/1, Relational Operator9/1, Relational Operator3/1
  Gain/1 -> Product1/2, Product1/1, Product/2
  Saturation1/1 -> Divide1/3
  Relational Operator12/1 -> Logical Operator4/1
  Saturation/1 -> Divide/2
  [VehSpeed_mps] -> Saturation/1
  [TargetExist] -> TargetExist/1
  [TargetExist2] -> TargetExist2/1
  Object/1 -> Bus Selector3/1
  Bus Selector3/1 -> [x_raw]  "<x>"
  Bus Selector3/2 -> [vx_raw]  "<vx>"
  Bus Selector3/3 -> [ax_raw]  "<ax>"
  LC_Time/1 -> [LCTime]
  VehStatus/1 -> Bus Selector1/1
  Bus Selector1/1 -> [VehSpeed_mps]  "<vRef>"
  [id_raw] -> Switch3/3
  Relational Operator5/1 -> Logical Operator6/2
  [y_raw] -> Add7/1
  [LCTime] -> MinMax/2, Gain3/1
  Gain3/1 -> Add6/1
  [y_raw] -> Abs4/1
  Abs4/1 -> Relational Operator5/2
  Relational Operator8/1 -> Logical Operator6/1
  Constant9/1 -> MinMax/1
  MinMax/1 -> Divide2/2
  Divide2/1 -> Add7/2
  Abs5/1 -> Relational Operator8/1
  [vy_raw] -> Divide2/1
  Add6/1 -> Relational Operator5/1, Relational Operator8/2
  Constant10/1 -> Add6/2
  Switch3/1 -> [id]
  Add7/1 -> Abs5/1
  C/1 -> Switch3/1
  [x_raw] -> Abs2/1
  [id] -> Switch2/2, Switch4/2, Switch1/2
  [vx_raw] -> Gain2/1
  [ax_raw] -> Gain4/1
  Constant2/1 -> Switch2/3
  Constant36/1 -> Switch4/3
  Constant1/1 -> Switch1/3
  Bus Selector3/4 -> [y_raw]  "<y>"
  Bus Selector3/5 -> [vy_raw]  "<vy>"
  Logical Operator6/1 -> Switch3/2
  Bus Selector3/6 -> [id_raw]  "<id>"
  Switch1/1 -> [x]
  Switch2/1 -> [vx]
  Switch4/1 -> [ax]
  Abs2/1 -> Switch1/1
  Gain2/1 -> Switch2/1
  Gain4/1 -> Switch4/1

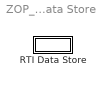
== system ZOP_Main/RTI Data/RTI Data Store/RTI Data Store ==
  RTI Data Store : Subsystem  mask(RTI_DATA_STORE){}
      mask help:
      | RTI Data Store Block. This block is used by RTI to store internal model dependent data. Deleting this block will result in data loss.
      |
      | NEVER DELETE, COPY, OR MODIFY THIS BLOCK!
      mask Help:
      | RTI Data Store Block. This block is used by RTI to store internal model dependent data. Deleting this block will result in data loss.
      | 
      | NEVER DELETE, COPY, OR MODIFY THIS BLOCK!
      mask Display: text(0.5, 0.5, ' ', 'HorizontalAlignment', 'center');

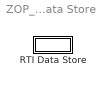
== system ZOP_Main/RTI Data/RTI Data Store/RTI Data Store/RTI Data Store ==
  RTI Data Store : Subsystem  mask(RTI_DATA_STORE){}
      mask help:
      | RTI Data Store Block. This block is used by RTI to store internal model dependent data. Deleting this block will result in data loss.
      |
      | NEVER DELETE, COPY, OR MODIFY THIS BLOCK!
      mask Help:
      | RTI Data Store Block. This block is used by RTI to store internal model dependent data. Deleting this block will result in data loss.
      | 
      | NEVER DELETE, COPY, OR MODIFY THIS BLOCK!
      mask Display: text(0.5, 0.5, ' ', 'HorizontalAlignment', 'center');

== system ZOP_Main/RTI Data/RTI Data Store/RTI Data Store/RTI Data Store/RTI Data Store ==

== stateflow chart ZOP_Main/Light_Process/Chart ==
  state Off
    en:
    Flag=0;
  state init
    en:
    Flag=0;
  state On
    du:
    Flag=1;
  (default) -> Off
  On -> Off : [dist < -5 || time < 0|| (traf_sign == 1 && dist <= 1)]
  Off -> init : [time > 0 && dist > 0]
  init -> On : [time > 0 && dist > 0 && dist / (velocity + 0.0001) <= 5]
  data: dist input; velocity input; Flag output; time input; traf_sign input
